simulink model "ex4"  (R2025b)
settings: Solver=VariableStepAuto  StartTime=0.0  StopTime=10.0  RelTol=1e-3
settings Model: Creator=vladl  LastModifiedBy=vladl

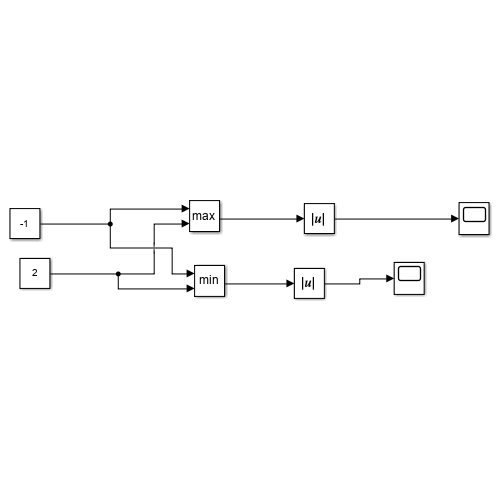
[thumbnail: Simulink's stored preview of the top-level diagram]
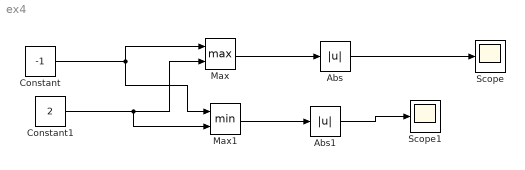
== system ex4 ==
  Abs : Abs  SaturateOnIntegerOverflow=off
  Abs1 : Abs  SaturateOnIntegerOverflow=off
  Constant : Constant  Value=-1
  Constant1 : Constant  Value=2
  Max : MinMax  Function=max  Inputs=2
  Max1 : MinMax  Inputs=2
  Scope : Scope
      settings: ActiveDisplayYMinimum=1  ActiveDisplayYMaximum=3
  Scope1 : Scope
      settings: ActiveDisplayYMinimum=0.9  ActiveDisplayYMaximum=1.1
  wires:
  Constant/1 -> Max1/1, Max/1
  Constant1/1 -> Max/2, Max1/2
  Max1/1 -> Abs1/1
  Abs1/1 -> Scope1/1
  Max/1 -> Abs/1
  Abs/1 -> Scope/1
